simulink model "decharge"  (R2020a)
settings: Solver=VariableStepAuto  StartTime=0.0  StopTime=5000  RelTol=1e-3
undefined symbols (not defined in the file): Ion, Lithium
libraries: powerlib x13, electricdrivelib x2
settings Model: Creator=guill  LastModifiedBy=guill

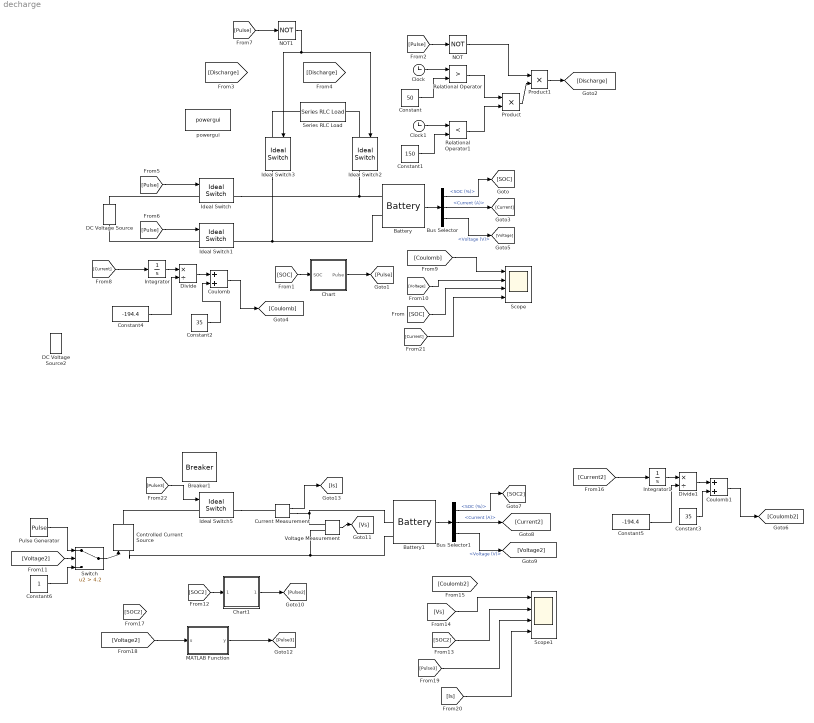
== system decharge ==
  Battery : electricdrivelib/Extra Sources/Battery  BatType=Lithium-Ion  ShowTempParam=off  ThermalPreset=no  ShowAgeParam=off  NomV=3.8  NomQ=5.4  SOC=35  Batt_Tr=30  PresetModel=off  MaxQ=5.4  MinV=3.3  FullV=4.2  Dis_rate=2.3478  R=0.007037  Normal_OP=4.8835  expZone="[4.1055      0.2653]"  current=[6.5 13 32.5]  Units=Time  Tci=20  NomT=20  T2=-30  MaxQ2=4.8  FullV2=7.1  Normal_OP2=5.655  expZone2="[6.58           1]"  Rca=0.6  ti=2000  Dp=0  Neq0=0  Tsim=1e6  Ta1=25  Qeol=5.4*0.9  Reol=0.013333*1.2  Char_age=[2.3478, 3]  Dis_age=[2.3478, 10]  N1=1500  N2=10500  N3=1000  N4=1400  Ta2=45  N5=950
  Battery1 : electricdrivelib/Extra Sources/Battery  BatType=Lithium-Ion  ShowTempParam=on  ThermalPreset="3.6V  2.0Ah"  ShowAgeParam=off  NomV=3.5  NomQ=2  SOC=35  Batt_Tr=30  PresetModel=off  MaxQ=2.05  MinV=2.625  FullV=4.1  Dis_rate=0.4  R=0.017  Normal_OP=1.8087  expZone="[3.88         0.2]"  current=[6.5 13 32.5]  Units=Time  Tci=20  NomT=115  T2=0  MaxQ2=1.65  FullV2=4  Normal_OP2=3.25  expZone2="[3.8         0.2]"  Rca=0.06  ti=1000  Dp=0  Neq0=0  Tsim=1e6  Ta1=25  Qeol=5.4*0.9  Reol=0.013333*1.2  Char_age=[2.3478, 3]  Dis_age=[2.3478, 10]  N1=1500  N2=10500  N3=1000  N4=1400  Ta2=45  N5=950
  Breaker1 : powerlib/Elements/Breaker  InitialState=0  SwitchingTimes="[1/60  5/60]"  External=on  BreakerResistance=0.01  SnubberResistance=1e6  SnubberCapacitance=inf  Measurements=None  MoreParameters=on  NoBreakLoop=off
  Bus Selector : BusSelector  OutputSignals=SOC (%),Current (A),Voltage (V)
  Bus Selector1 : BusSelector  OutputSignals=SOC (%),Current (A),Voltage (V)
  Chart : Stateflow chart  TreatAsAtomicUnit=on
  Chart1 : Stateflow chart  TreatAsAtomicUnit=on
  Clock : Clock
  Clock1 : Clock
  Constant : Constant  Value=50
  Constant1 : Constant  Value=150
  Constant2 : Constant  Value=35
  Constant3 : Constant  Value=35
  Constant4 : Constant  Value=-194.4
  Constant5 : Constant  Value=-194.4
  Constant6 : Constant
  Controlled Current Source : powerlib/Electrical Sources/Controlled Current Source  Initialize=on  Source_Type=AC  Amplitude=0  Phase=0  Frequency=0  Measurements=None
  Coulomb : Sum
  Coulomb1 : Sum
  Current Measurement : powerlib/Measurements/Current Measurement  PhasorSimulation=off  OutputType=Complex  PSBequivalent=0
  DC Voltage Source : powerlib/Electrical Sources/DC Voltage Source  Amplitude=7.6  Measurements=None
  DC Voltage Source2 : powerlib/Electrical Sources/DC Voltage Source  Amplitude=4.2  Measurements=None
  Divide : Product  Inputs=*/
  Divide1 : Product  Inputs=*/
  Ideal Switch{,1..3,5} (5 alike) : powerlib/Power Electronics/Ideal Switch  Ron=0.001  Lon=0  IC=0  Rs=1e5  Cs=inf  Measurements=on
  Integrator : Integrator
  Integrator1 : Integrator
  MATLAB Function : MATLAB Function  TreatAsAtomicUnit=on
  NOT : Logic  Operator=NOT  IconShape=distinctive  AllPortsSameDT=off  OutDataTypeStr=boolean
  NOT1 : Logic  Operator=NOT  IconShape=distinctive  AllPortsSameDT=off  OutDataTypeStr=boolean
  Product : Product
  Product1 : Product
  Pulse Generator : DiscretePulseGenerator  PulseType=Time based  Period=1  PulseWidth=5
  Relational Operator : RelationalOperator  Operator=>  OutDataTypeStr=boolean  RndMeth=Simplest
  Relational Operator1 : RelationalOperator  Operator=<  OutDataTypeStr=boolean  RndMeth=Simplest
  Scope : Scope  NumInputPorts=4
  Scope1 : Scope  NumInputPorts=4
  Series RLC Load : powerlib/Elements/Series RLC Load  LConnTagsString=a  RConnTagsString=__new0  NominalVoltage=10  NominalFrequency=60  ActivePower=1000  InductivePower=0  CapacitivePower=0  Setx0=off  InitialVoltage=0  SetiL0=off  InitialCurrent=0  Measurements=None  LoadType=constant Z
  Switch : Switch  Criteria=u2 > Threshold  Threshold=4.2  ZeroCross=off
  Voltage Measurement : powerlib/Measurements/Voltage Measurement  PhasorSimulation=off  OutputType=Complex  PSBequivalent=0
  powergui : powerlib/powergui  Priority=1  SimulationMode=Continuous  SampleTime=50e-6  frequency=60  Iterations=50  frequencyindice=0  Pbase=100e6  ErrMax=1e-4  UnitsV=kV  UnitsW=MW  buscounter=0  FunctionMessages=off  echomessages=off  EnableUseOfTLC=off  CurrentSourceSwitches=off  DisableSnubberDevices=off  DisableRonSwitches=off  DisableVfSwitches=off  DisplayEquations=off  AutomaticDiscreteSolvers=off  SolverType=Tustin/Backward Euler (TBE)  Interpol=off  ExternalGateDelay=off  methode=off  Ts=100  x0status=blocks  SPID=on  SwTol=0  HookPort=off  NonlinearTolerance=1e-4  nMaxIteration=100  ContinueOnMaxIteration=off  RestoreLinks=warning  ResistiveCurrentMeasurement=off  Frange=[0:2:500]  Ylog=off  Xlog=on  ShowGrid=off  save=off  variable=ZData  structure=0  ZoomFFT=off  StartTime=0.0  cycles=1  DisplayStyle=1  fundamental=60  FreqAxis=off  MaxFrequency=1000  frequencyindicesteady=1  RmsSteady=1  display=off
  wires:
  Battery/1 -> Bus Selector/1
  Bus Selector/1 -> [SOC]  "<SOC (%)>"
  [SOC] -> Chart/1(SOC)
  Chart/1(Pulse) -> [Pulse]
  [Pulse] -> NOT/1
  Clock/1 -> Relational Operator/1
  Constant/1 -> Relational Operator/2
  Clock1/1 -> Relational Operator1/1
  Constant1/1 -> Relational Operator1/2
  Relational Operator1/1 -> Product/2
  Relational Operator/1 -> Product/1
  Product/1 -> Product1/2
  NOT/1 -> Product1/1
  Product1/1 -> [Discharge]
  [Pulse] -> Ideal Switch1/1
  [Pulse] -> Ideal Switch/1
  [Pulse] -> NOT1/1
  NOT1/1 -> Ideal Switch2/1, Ideal Switch3/1
  Bus Selector/2 -> [Current]  "<Current (A)>"
  [Current] -> Integrator/1
  [Coulomb] -> Scope/1
  Integrator/1 -> Divide/1
  Constant4/1 -> Divide/2
  Divide/1 -> Coulomb/1
  Constant2/1 -> Coulomb/2
  Coulomb/1 -> [Coulomb]
  Bus Selector/3 -> [Voltage]  "<Voltage (V)>"
  [SOC] -> Scope/3
  [Voltage] -> Scope/2
  Bus Selector1/3 -> [Voltage2]  "<Voltage (V)>"
  Bus Selector1/2 -> [Current2]  "<Current (A)>"
  Bus Selector1/1 -> [SOC2]  "<SOC (%)>"
  Battery1/1 -> Bus Selector1/1
  Coulomb1/1 -> [Coulomb2]
  Constant3/1 -> Coulomb1/2
  Divide1/1 -> Coulomb1/1
  Constant5/1 -> Divide1/2
  Integrator1/1 -> Divide1/1
  [Current2] -> Integrator1/1
  Chart1/1(Pulse2) -> [Pulse2]
  [SOC2] -> Chart1/1(SOC2)
  Voltage Measurement/1 -> [Vs]
  [Vs] -> Scope1/1
  [SOC2] -> Scope1/2
  [Voltage2] -> MATLAB Function/1(u)
  MATLAB Function/1(y) -> [Pulse3]
  [Pulse3] -> Scope1/3
  Current Measurement/1 -> [Is]
  [Is] -> Scope1/4
  [Current] -> Scope/4
  [Pulse3] -> Ideal Switch5/1
  Switch/1 -> Controlled Current Source/1
  [Voltage2] -> Switch/2
  Pulse Generator/1 -> Switch/1
  Constant6/1 -> Switch/3
  connections:
  Battery/LConn2 -- Ideal Switch3/RConn1 -- Ideal Switch1/RConn1
  Ideal Switch/RConn1 -- Ideal Switch2/RConn1 -- Battery/LConn1
  Series RLC Load/LConn1 -- Ideal Switch3/LConn1
  Ideal Switch2/LConn1 -- Series RLC Load/RConn1
  Voltage Measurement/LConn1 -- Current Measurement/RConn1 -- Battery1/LConn1
  Battery1/LConn2 -- Controlled Current Source/LConn1 -- Voltage Measurement/LConn2
  DC Voltage Source/RConn1 -- Ideal Switch/LConn1
  Ideal Switch1/LConn1 -- DC Voltage Source/LConn1
  Ideal Switch5/RConn1 -- Current Measurement/LConn1
  Ideal Switch5/LConn1 -- Controlled Current Source/RConn1

== matlab function decharge/MATLAB Function ==
  data: u input; y output
function y = fcn(u)
Pulse=1;
if u>3.6 && u<4.2
    Pulse=0;
else
    Pulse=1
end
y=Pulse;
end

== stateflow chart decharge/Chart ==
  state Charge
    entry: Pulse=1
  state Discharge
    entry: Pulse=0
  (default) -> Charge
  Charge -> Discharge : [SOC>80]
  Discharge -> Charge : [SOC<40]
  data: SOC input; Pulse output

== stateflow chart decharge/Chart1 ==
  state Charge2
    entry: Pulse2=1
  state Discharge2
    entry: Pulse2=0
  (default) -> Charge2
  Charge2 -> Discharge2 : [SOC2>80]
  Discharge2 -> Charge2 : [SOC2<75]
  data: SOC2 input; Pulse2 output
